simulink model "apcex1"  (Simulink 3.00)
settings: Solver=ode45  SolverMode=SingleTasking  StartTime=0.0  StopTime=3  RelTol=1e-3  AbsTol=1e-6
settings Model: OptimizeBlockIOStorage=off

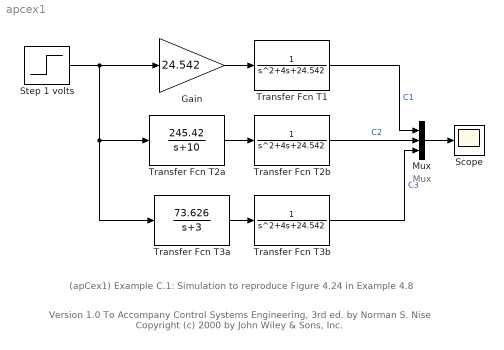
== system apcex1 ==
  note: Mux
  note: (apCex1) Example C.1: Simulation to reproduce Figure 4.24 in Example 4.8
  note: Version 1.0
      | To Accompany Control Systems Engineering, 3rd ed. by Norman S. Nise
      | Copyright (c) 2000 by John Wiley & Sons, Inc.
  Gain : Gain  Gain=24.542  SaturateOnIntegerOverflow=on
  Mux : Mux  Inputs=3
  Scope : Scope
      settings: TimeRange=auto  YMin=0  YMax=2  SaveToWorkspace=off  SaveName=ScopeData  DataFormat=Matrix
  "Step 1 volts " : Step  Time=0  Before=0  After=1  SampleTime=0
  Transfer Fcn T1 : TransferFcn  Numerator=1  Denominator=[1 4 24.542]
  Transfer Fcn T2a : TransferFcn  Numerator=245.42  Denominator=[1 10]
  Transfer Fcn T2b : TransferFcn  Numerator=1  Denominator=[1 4 24.542]
  Transfer Fcn T3a : TransferFcn  Numerator=73.626  Denominator=[1 3]
  Transfer Fcn T3b : TransferFcn  Numerator=1  Denominator=[1 4 24.542]
  wires:
  Transfer Fcn T2a/1 -> Transfer Fcn T2b/1
  Transfer Fcn T3a/1 -> Transfer Fcn T3b/1
  "Step 1 volts "/1 -> Transfer Fcn T3a/1, Transfer Fcn T2a/1, Gain/1
  Gain/1 -> Transfer Fcn T1/1
  Transfer Fcn T1/1 -> Mux/1  "C1"
  Transfer Fcn T2b/1 -> Mux/2  "C2"
  Transfer Fcn T3b/1 -> Mux/3  "C3"
  Mux/1 -> Scope/1
